simulink model "ImpMinJerkTraj"  (R2025b)
settings: Solver=FixedStepAuto  StartTime=0.0  StopTime=inf  FixedStep=Ts  RelTol=1e-3
model workspace (MAT data in the model file):
  SL_ROS_VariableLengthArrays_MaxSizes.CommonInfo.ArrayTruncateAction = 'EmitWarning'
  SL_ROS_VariableLengthArrays_MaxSizes.MsgTypeMap = containers.Map
  SL_ROS_VariableLengthArrays_MaxSizes.MsgTypeMap.serialization.keys = {'sensor_msgs/JointState'}
  SL_ROS_VariableLengthArrays_MaxSizes.MsgTypeMap.serialization.values{1}(1).PropertyName = 'effort'
  SL_ROS_VariableLengthArrays_MaxSizes.MsgTypeMap.serialization.values{1}(1).DataType = 'double'
  SL_ROS_VariableLengthArrays_MaxSizes.MsgTypeMap.serialization.values{1}(1).MaxLength = 3
  SL_ROS_VariableLengthArrays_MaxSizes.MsgTypeMap.serialization.values{1}(2).PropertyName = 'name'
  SL_ROS_VariableLengthArrays_MaxSizes.MsgTypeMap.serialization.values{1}(2).DataType = 'std_msgs/String'
  SL_ROS_VariableLengthArrays_MaxSizes.MsgTypeMap.serialization.values{1}(2).MaxLength = 16
  SL_ROS_VariableLengthArrays_MaxSizes.MsgTypeMap.serialization.values{1}(3).PropertyName = 'position'
  SL_ROS_VariableLengthArrays_MaxSizes.MsgTypeMap.serialization.values{1}(3).DataType = 'double'
  SL_ROS_VariableLengthArrays_MaxSizes.MsgTypeMap.serialization.values{1}(3).MaxLength = 3
  SL_ROS_VariableLengthArrays_MaxSizes.MsgTypeMap.serialization.values{1}(4).PropertyName = 'velocity'
  SL_ROS_VariableLengthArrays_MaxSizes.MsgTypeMap.serialization.values{1}(4).DataType = 'double'
  SL_ROS_VariableLengthArrays_MaxSizes.MsgTypeMap.serialization.values{1}(4).MaxLength = 3
  SL_ROS_VariableLengthArrays_MaxSizes.MsgTypeMap.serialization.uniformity = 0
  SL_ROS_VariableLengthArrays_MaxSizes.MsgTypeMap.serialization.keyType = 'char'
  SL_ROS_VariableLengthArrays_MaxSizes.MsgTypeMap.serialization.valueType = 'any'
values from neighbouring files (symbols this model uses):
  hiddenLayerSizeCtrl = 20    [InitMinJerkTraj.m]
  hiddenLayerSizeObsv = 5    [InitMinJerkTraj.m]
  p = 3    [InitMinJerkTraj.m]
  timePoints = [0, 12, 27, 44, 60]    [InitMinJerkTraj.m]
  torque2voltage = voltage_max ./ u_max    [InitMinJerkTraj.m]
  u_max = motor_max_torque * gear_ratio    [InitMinJerkTraj.m]
  u_min = - motor_max_torque * gear_ratio    [InitMinJerkTraj.m]
  Vctrl0 = 0.1 * randn(hiddenLayerSizeCtrl, inputLayerSizeCtrl)    [InitMinJerkTraj.m]
  Vobsv0 = 0.1 * randn(hiddenLayerSizeObsv, inputLayerSizeObsv)    [InitMinJerkTraj.m]
  wayPoints = [q1WayPoints; q2WayPoints; q3WayPoints]    [InitMinJerkTraj.m]
  Wctrl0 = 0.1 * randn(outputLayerSizeCtrl, hiddenLayerSizeCtrl)    [InitMinJerkTraj.m]
  Wobsv0 = 0.1 * randn(outputLayerSizeObsv, hiddenLayerSizeObsv)    [InitMinJerkTraj.m]
  x_hat0 = zeros(n, 1)    [InitMinJerkTraj.m]
undefined symbols (not defined in the file or in its folder): effort, effort_SL_Info, position, position_SL_Info
libraries: ros2lib x3, slpidlib x3, shareduavrstlib x1
settings Model: Creator=Asus  LastModifiedBy=Asus
settings OptimizationCC: DefaultParameterBehavior=Inlined  EnhancedBackFolding=on  PassReuseOutputArgsAs=Individual arguments  ZeroExternalMemoryAtStartup=off  ZeroInternalMemoryAtStartup=off  MaxStackSize=64  OptimizeBlockOrder=speed  DifferentSizesBufferReuse=on  OptimizationCustomize=off  EfficientTunableParamExpr=on
settings DebuggingCC: ParameterTunabilityLossMsg=error
settings SFSimCC: MATLABDynamicMemAlloc=off
settings RTWCC: SystemTargetFile=ert.tlc  HardwareBoard=Robot Operating System 2 (ROS 2)  TLCOptions="-aInlineSetEventsForThisBaseRateFcn=TLC_FALSE -aSuppressMultiTaskScheduler=TLC_FALSE  -aRateBasedStepFcn=0"  TemplateMakefile=ert_default_tmf  Toolchain=Colcon Tools  TargetLang=C++  Description=Embedded Coder
settings CodeAppCC: ForceParamTrailComments=on  IgnoreCustomStorageClasses=off  MaxIdLength=95.0  OperatorAnnotations=on  SimulinkDataObjDesc=on  SFDataObjDesc=on  InsertBlockDesc=on
settings ERTTargetCC: RootIOFormat=Structure reference  CodeInterfacePackaging=C++ class

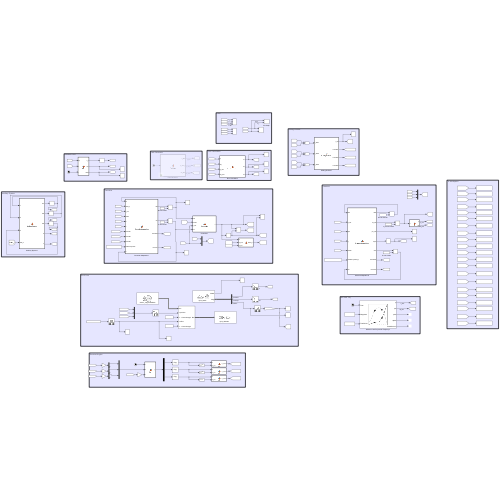
[thumbnail: Simulink's stored preview of the top-level diagram]
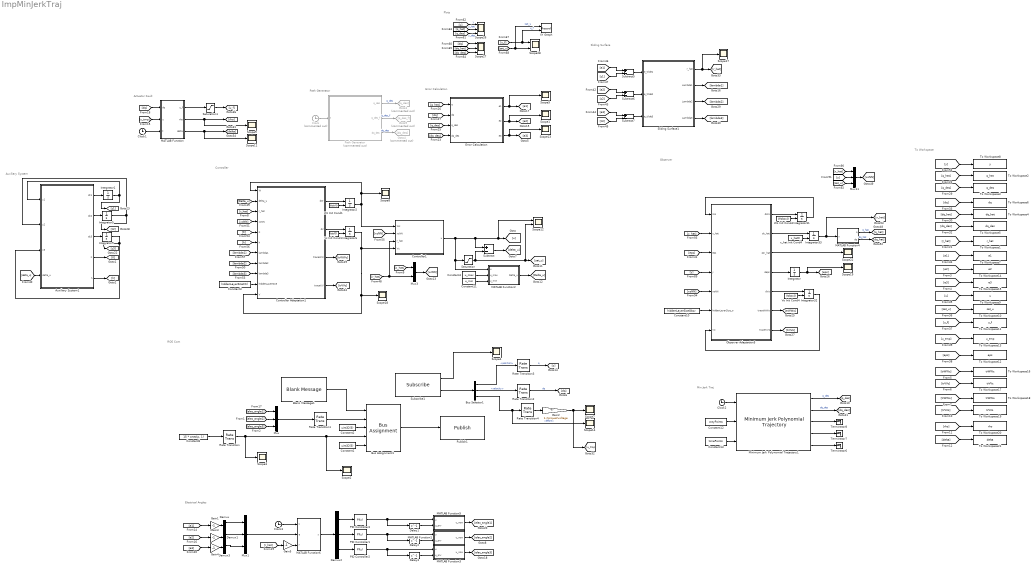
== system ImpMinJerkTraj ==
  note: To Workspace
  note: Electrical Angles
  note: Plots
  note: Path Generator
  note: Observer
  note: ROS Com
  note: Actuator Fault
  note: Min Jerk Traj
  note: Auxiliary System
  note: Error Calculation
  note: Sliding Surface
  note: Controller
  Auxiliary System1 : MATLAB Function  TreatAsAtomicUnit=on
  Blank Message1 : ros2lib/Blank Message  messageClass=Message  entityType=sensor_msgs/JointState  messageType=sensor_msgs/JointState  SampleTime=0.02
  Bus Assignment1 : BusAssignment  AssignedSignals=position,position_SL_Info.CurrentLength,effort,effort_SL_Info.CurrentLength
  Bus Selector1 : BusSelector  OutputSignals=position,velocity,effort
  Clock : Clock  Commented=on
  Clock1 : Clock
  Clock2 : Clock
  Clock3 : Clock
  Constant1 : Constant  Value=uint32(3)
  Constant10 : Constant  Value=hiddenLayerSizeObsv
  Constant11 : Constant  Value=u_min
  Constant12 : Constant  Value=wayPoints
  Constant13 : Constant  Value=timePoints
  Constant2 : Constant  Value=uint32(3)
  Constant3 : Constant  Value=hiddenLayerSizeCtrl
  Constant4 : Constant  Value=u_max
  Constant8 : Constant  Value=15 * ones(p, 1)
  Controller Adaptation1 : MATLAB Function  TreatAsAtomicUnit=on
  Controller1 : MATLAB Function  TreatAsAtomicUnit=on
  Delay1 : Delay  DelayLength=1  InitialCondition=0
  Delay2 : Delay  DelayLength=1  InitialCondition=0
  Delay3 : Delay  DelayLength=1  InitialCondition=0
  Demux : Demux  Outputs=2
  Demux1 : Demux  Outputs=2
  Demux2 : Demux  Outputs=3
  Demux3 : Demux  Outputs=2
  Error Calculation : MATLAB Function  TreatAsAtomicUnit=on
  Gain{1,3..5} (4 alike) : Gain  Gain=-1
  Gain2 : Gain  Gain=1./torque2voltage
  Goto3 : Goto  Commented=on  GotoTag=q_des
  Goto4 : Goto  Commented=on  GotoTag=dq_des
  Goto9 : Goto  Commented=on  GotoTag=q_des_f
  Integrator : Integrator  InitialCondition=5 * ones(p, 1)
  Integrator1 : Integrator  InitialCondition=zeros(2, 1)
  Integrator{2,6,31..33} (5 alike) : Integrator  InitialConditionSource=external  InitialCondition=[0.5; 0.5]
  Integrator5 : Integrator  InitialCondition=zeros(2, 1)
  Integrator9 : Integrator  InitialCondition=zeros(2, 1)
  MATLAB Function : MATLAB Function  TreatAsAtomicUnit=on
  MATLAB Function1 : MATLAB Function  TreatAsAtomicUnit=on
  MATLAB Function2 : MATLAB Function  TreatAsAtomicUnit=on
  MATLAB Function3 : MATLAB Function  TreatAsAtomicUnit=on
  MATLAB Function4 : MATLAB Function  TreatAsAtomicUnit=on
  MATLAB Function5 : MATLAB Function  TreatAsAtomicUnit=on
  MATLAB Function6 : MATLAB Function  TreatAsAtomicUnit=on
  Minimum Jerk Polynomial Trajectory1 : shareduavrstlib/Minimum Jerk Polynomial Trajectory  ShowBCInputPort=off  ShowPolynomialCoefs=off  ShowStatusOutputPort=off  TimeAllocation=off  TimeWeight=100  MinSegmentTime=0.1  MaxSegmentTime=1  MaxIteration=1500  MaxTime=10  SimulateUsing=Interpreted execution
      settings: LibrarySourceBlock=robotutilslib/Minimum Jerk Polynomial Trajectory
  Mux : Mux  Inputs=3
  Mux1 : Mux  Inputs=3
  Mux11 : Mux  Inputs=3
  Mux3 : Mux  Inputs=2
  Observer Adaptation5 : MATLAB Function  TreatAsAtomicUnit=on
  PID Controller1 : slpidlib/PID Controller  Controller=PI  Form=Parallel  TimeDomain=Discrete-time  UseExternalTs=off  SampleTime=-1  IntegratorMethod=Trapezoidal  FilterMethod=Forward Euler  ControllerParametersSource=internal  P=0.01  I=20  UseKiTs=off  D=0  UseExternalDerivativeSource=off  N=100  UseFilter=on  TunerSelectOption=Transfer Function Based (PID Tuner App)  InitialConditionSource=internal  InitialConditionForIntegrator=0  InitialConditionForFilter=0  DifferentiatorICPrevScaledInput=0  ExternalReset=none  TrackingMode=off  Kt=1  LimitOutput=off  SatLimitsSource=internal  UpperSaturationLimit=50  LowerSaturationLimit=-50  LinearizeAsGain=on  AntiWindupMode=none  Kb=1  LimitIntegrator=off  UpperIntegratorSaturationLimit=50  LowerIntegratorSaturationLimit=-50  POutMin=[]  POutMax=[]  IOutMin=[]  IOutMax=[]  DOutMin=[]  DOutMax=[]  NOutMin=[]  NOutMax=[]  SumOutMin=[]  SumOutMax=[]  SaturationOutMin=[]  SaturationOutMax=[]  PParamMin=[]  PParamMax=[]  IParamMin=[]  IParamMax=[]  DParamMin=[]  DParamMax=[]  NParamMin=[]  NParamMax=[]  KbParamMin=[]  KbParamMax=[]  KtParamMin=[]  KtParamMax=[]  KbOutMin=[]  KbOutMax=[]  KtOutMin=[]  KtOutMax=[]  IntegratorOutMin=[]  IntegratorOutMax=[]  FilterOutMin=[]  FilterOutMax=[]  SumI1OutMin=[]  SumI1OutMax=[]  SumI2OutMin=[]  SumI2OutMax=[]  SumI3OutMin=[]  SumI3OutMax=[]  SumI4OutMin=[]  SumI4OutMax=[]  SumDOutMin=[]  SumDOutMax=[]  DifferentiatorOutMin=[]  DifferentiatorOutMax=[]  FilterDiffOutCoefMin=[]  FilterDiffOutCoefMax=[]  ReciprocalOutMin=[]  ReciprocalOutMax=[]  SumDenOutMin=[]  SumDenOutMax=[]  SumNumOutMin=[]  SumNumOutMax=[]  DivideOutMin=[]  DivideOutMax=[]  UdiffTsProdOutMin=[]  UdiffTsProdOutMax=[]  NTsProdOutMin=[]  NTsProdOutMax=[]  UintegralTsProdOutMin=[]  UintegralTsProdOutMax=[]  UngainTsProdOutMin=[]  UngainTsProdOutMax=[]  ClampingZeroOutDataTypeStr=Inherit: Inherit via back propagation  ClampingZeroOutMin=[]  ClampingZeroOutMax=[]  FilterDenConstantOutDataTypeStr=Inherit: Inherit via back propagation  FilterDenConstantOutMin=[]  FilterDenConstantOutMax=[]  PCopyOutDataTypeStr=Inherit: Inherit via back propagation  PCopyOutMin=[]  PCopyOutMax=[]  NCopyOutDataTypeStr=Inherit: Inherit via back propagation  NCopyOutMin=[]  NCopyOutMax=[]  IntegratorContinuousStateAttributes=''  IntegratorStateMustResolveToSignalObject=off  IntegratorRTWStateStorageClass=Auto  FilterContinuousStateAttributes=''  FilterStateMustResolveToSignalObject=off  FilterRTWStateStorageClass=Auto  ParallelPVariant=InternalParameters  IdealPVariant=Disabled  IVariant=InternalParameters  DVariant=Disabled  IntegratorVariant=Discrete  SatVariant=Disabled  AWVariant=Passthrough  PCopyVariant=Disabled  TRVariant=Disabled  FdbkBlocksVariant=Forward  IdealPFdbkVariant=Disabled  SatFdbkVariant=Disabled  DerivativeFilterVariant=Disabled  NVariant=Disabled  NCopyVariant=Disabled_SignalSpec  FilterICVariant=Disabled  IntegratorICVariant=InternalICs  ExternalResetVariant=Disabled  TRSumVariant=Passthrough  SumFdbkVariant=Disabled  SumVariant=Sum_PI  TsampFilterVariant=InternalTs  TsampNgainVariant=Passthrough  TsampIntegralVariant=Disabled_SignalSpec  ExternalSaturationOutDataTypeStr=Inherit: Same as second input  DerivativeSourceVariant=Disabled  PreIntVariant=InternalPreInt
  PID Controller2 : slpidlib/PID Controller  Controller=PI  Form=Parallel  TimeDomain=Discrete-time  UseExternalTs=off  SampleTime=-1  IntegratorMethod=Trapezoidal  FilterMethod=Forward Euler  ControllerParametersSource=internal  P=0.01  I=20  UseKiTs=off  D=0  UseExternalDerivativeSource=off  N=100  UseFilter=on  TunerSelectOption=Transfer Function Based (PID Tuner App)  InitialConditionSource=internal  InitialConditionForIntegrator=0  InitialConditionForFilter=0  DifferentiatorICPrevScaledInput=0  ExternalReset=none  TrackingMode=off  Kt=1  LimitOutput=off  SatLimitsSource=internal  UpperSaturationLimit=50  LowerSaturationLimit=-50  LinearizeAsGain=on  AntiWindupMode=none  Kb=1  LimitIntegrator=off  UpperIntegratorSaturationLimit=50  LowerIntegratorSaturationLimit=-50  POutMin=[]  POutMax=[]  IOutMin=[]  IOutMax=[]  DOutMin=[]  DOutMax=[]  NOutMin=[]  NOutMax=[]  SumOutMin=[]  SumOutMax=[]  SaturationOutMin=[]  SaturationOutMax=[]  PParamMin=[]  PParamMax=[]  IParamMin=[]  IParamMax=[]  DParamMin=[]  DParamMax=[]  NParamMin=[]  NParamMax=[]  KbParamMin=[]  KbParamMax=[]  KtParamMin=[]  KtParamMax=[]  KbOutMin=[]  KbOutMax=[]  KtOutMin=[]  KtOutMax=[]  IntegratorOutMin=[]  IntegratorOutMax=[]  FilterOutMin=[]  FilterOutMax=[]  SumI1OutMin=[]  SumI1OutMax=[]  SumI2OutMin=[]  SumI2OutMax=[]  SumI3OutMin=[]  SumI3OutMax=[]  SumI4OutMin=[]  SumI4OutMax=[]  SumDOutMin=[]  SumDOutMax=[]  DifferentiatorOutMin=[]  DifferentiatorOutMax=[]  FilterDiffOutCoefMin=[]  FilterDiffOutCoefMax=[]  ReciprocalOutMin=[]  ReciprocalOutMax=[]  SumDenOutMin=[]  SumDenOutMax=[]  SumNumOutMin=[]  SumNumOutMax=[]  DivideOutMin=[]  DivideOutMax=[]  UdiffTsProdOutMin=[]  UdiffTsProdOutMax=[]  NTsProdOutMin=[]  NTsProdOutMax=[]  UintegralTsProdOutMin=[]  UintegralTsProdOutMax=[]  UngainTsProdOutMin=[]  UngainTsProdOutMax=[]  ClampingZeroOutDataTypeStr=Inherit: Inherit via back propagation  ClampingZeroOutMin=[]  ClampingZeroOutMax=[]  FilterDenConstantOutDataTypeStr=Inherit: Inherit via back propagation  FilterDenConstantOutMin=[]  FilterDenConstantOutMax=[]  PCopyOutDataTypeStr=Inherit: Inherit via back propagation  PCopyOutMin=[]  PCopyOutMax=[]  NCopyOutDataTypeStr=Inherit: Inherit via back propagation  NCopyOutMin=[]  NCopyOutMax=[]  IntegratorContinuousStateAttributes=''  IntegratorStateMustResolveToSignalObject=off  IntegratorRTWStateStorageClass=Auto  FilterContinuousStateAttributes=''  FilterStateMustResolveToSignalObject=off  FilterRTWStateStorageClass=Auto  ParallelPVariant=InternalParameters  IdealPVariant=Disabled  IVariant=InternalParameters  DVariant=Disabled  IntegratorVariant=Discrete  SatVariant=Disabled  AWVariant=Passthrough  PCopyVariant=Disabled  TRVariant=Disabled  FdbkBlocksVariant=Forward  IdealPFdbkVariant=Disabled  SatFdbkVariant=Disabled  DerivativeFilterVariant=Disabled  NVariant=Disabled  NCopyVariant=Disabled_SignalSpec  FilterICVariant=Disabled  IntegratorICVariant=InternalICs  ExternalResetVariant=Disabled  TRSumVariant=Passthrough  SumFdbkVariant=Disabled  SumVariant=Sum_PI  TsampFilterVariant=InternalTs  TsampNgainVariant=Passthrough  TsampIntegralVariant=Disabled_SignalSpec  ExternalSaturationOutDataTypeStr=Inherit: Same as second input  DerivativeSourceVariant=Disabled  PreIntVariant=InternalPreInt
  PID Controller4 : slpidlib/PID Controller  Controller=PI  Form=Parallel  TimeDomain=Discrete-time  UseExternalTs=off  SampleTime=-1  IntegratorMethod=Trapezoidal  FilterMethod=Forward Euler  ControllerParametersSource=internal  P=0.01  I=20  UseKiTs=off  D=0  UseExternalDerivativeSource=off  N=100  UseFilter=on  TunerSelectOption=Transfer Function Based (PID Tuner App)  InitialConditionSource=internal  InitialConditionForIntegrator=0  InitialConditionForFilter=0  DifferentiatorICPrevScaledInput=0  ExternalReset=none  TrackingMode=off  Kt=1  LimitOutput=off  SatLimitsSource=internal  UpperSaturationLimit=50  LowerSaturationLimit=-50  LinearizeAsGain=on  AntiWindupMode=none  Kb=1  LimitIntegrator=off  UpperIntegratorSaturationLimit=50  LowerIntegratorSaturationLimit=-50  POutMin=[]  POutMax=[]  IOutMin=[]  IOutMax=[]  DOutMin=[]  DOutMax=[]  NOutMin=[]  NOutMax=[]  SumOutMin=[]  SumOutMax=[]  SaturationOutMin=[]  SaturationOutMax=[]  PParamMin=[]  PParamMax=[]  IParamMin=[]  IParamMax=[]  DParamMin=[]  DParamMax=[]  NParamMin=[]  NParamMax=[]  KbParamMin=[]  KbParamMax=[]  KtParamMin=[]  KtParamMax=[]  KbOutMin=[]  KbOutMax=[]  KtOutMin=[]  KtOutMax=[]  IntegratorOutMin=[]  IntegratorOutMax=[]  FilterOutMin=[]  FilterOutMax=[]  SumI1OutMin=[]  SumI1OutMax=[]  SumI2OutMin=[]  SumI2OutMax=[]  SumI3OutMin=[]  SumI3OutMax=[]  SumI4OutMin=[]  SumI4OutMax=[]  SumDOutMin=[]  SumDOutMax=[]  DifferentiatorOutMin=[]  DifferentiatorOutMax=[]  FilterDiffOutCoefMin=[]  FilterDiffOutCoefMax=[]  ReciprocalOutMin=[]  ReciprocalOutMax=[]  SumDenOutMin=[]  SumDenOutMax=[]  SumNumOutMin=[]  SumNumOutMax=[]  DivideOutMin=[]  DivideOutMax=[]  UdiffTsProdOutMin=[]  UdiffTsProdOutMax=[]  NTsProdOutMin=[]  NTsProdOutMax=[]  UintegralTsProdOutMin=[]  UintegralTsProdOutMax=[]  UngainTsProdOutMin=[]  UngainTsProdOutMax=[]  ClampingZeroOutDataTypeStr=Inherit: Inherit via back propagation  ClampingZeroOutMin=[]  ClampingZeroOutMax=[]  FilterDenConstantOutDataTypeStr=Inherit: Inherit via back propagation  FilterDenConstantOutMin=[]  FilterDenConstantOutMax=[]  PCopyOutDataTypeStr=Inherit: Inherit via back propagation  PCopyOutMin=[]  PCopyOutMax=[]  NCopyOutDataTypeStr=Inherit: Inherit via back propagation  NCopyOutMin=[]  NCopyOutMax=[]  IntegratorContinuousStateAttributes=''  IntegratorStateMustResolveToSignalObject=off  IntegratorRTWStateStorageClass=Auto  FilterContinuousStateAttributes=''  FilterStateMustResolveToSignalObject=off  FilterRTWStateStorageClass=Auto  ParallelPVariant=InternalParameters  IdealPVariant=Disabled  IVariant=InternalParameters  DVariant=Disabled  IntegratorVariant=Discrete  SatVariant=Disabled  AWVariant=Passthrough  PCopyVariant=Disabled  TRVariant=Disabled  FdbkBlocksVariant=Forward  IdealPFdbkVariant=Disabled  SatFdbkVariant=Disabled  DerivativeFilterVariant=Disabled  NVariant=Disabled  NCopyVariant=Disabled_SignalSpec  FilterICVariant=Disabled  IntegratorICVariant=InternalICs  ExternalResetVariant=Disabled  TRSumVariant=Passthrough  SumFdbkVariant=Disabled  SumVariant=Sum_PI  TsampFilterVariant=InternalTs  TsampNgainVariant=Passthrough  TsampIntegralVariant=Disabled_SignalSpec  ExternalSaturationOutDataTypeStr=Inherit: Same as second input  DerivativeSourceVariant=Disabled  PreIntVariant=InternalPreInt
  Path Generator : MATLAB Function  Commented=on  TreatAsAtomicUnit=on
  Publish1 : ros2lib/Publish  topicSource=Specify your own  topic=/joint_desireds  messageType=sensor_msgs/JointState  QOSHistory=Keep last  QOSDepth=10  QOSReliability=Reliable  QOSDurability=Volatile  QOSDeadline=Inf  QOSLifespan=Inf  QOSLiveliness=Automatic  QOSLeaseDuration=Inf  QOSAvoidROSNamespaceConventions=off
  Rate Transition : RateTransition  OutPortSampleTime=0.02
  Rate Transition1 : RateTransition  OutPortSampleTime=0.02
  Rate Transition2 : RateTransition  OutPortSampleTime=Ts
  Rate Transition3 : RateTransition  OutPortSampleTime=Ts
  Rate Transition4 : RateTransition  OutPortSampleTime=Ts
  Saturation : Saturate  UpperLimit=u_max  LowerLimit=u_min
  Saturation1 : Saturate  UpperLimit=u_max  LowerLimit=u_min
  Scope{1..5,7..9,11,13..14,17..19,22} (15 alike) : Scope
      Scope1 settings: ActiveDisplayYMinimum=-0.24287807344006263  ActiveDisplayYMaximum=0.25287974310957717  DataLoggingVariableName=ScopeData3
      Scope11 settings: ActiveDisplayYMinimum=-1  ActiveDisplayYMaximum=1  DataLoggingVariableName=ScopeData6
      Scope13 settings: ActiveDisplayYMinimum=-0.29897924911149121  ActiveDisplayYMaximum=0.2090765790905024  DataLoggingVariableName=ScopeData13
      Scope14 settings: ActiveDisplayYMinimum=-12.649985074996948  ActiveDisplayYMaximum=12.652279615402222  DataLoggingVariableName=ScopeData14
      Scope17 settings: ActiveDisplayYMinimum=-9.1334368109122082  ActiveDisplayYMaximum=5.1770184739117182  DataLoggingVariableName=ScopeData19
      Scope18 settings: ActiveDisplayYMinimum=-1  ActiveDisplayYMaximum=1  DataLoggingVariableName=ScopeData10
      Scope19 settings: ActiveDisplayYMinimum=-0.056716812017258533  ActiveDisplayYMaximum=20.510451308155332  DataLoggingVariableName=ScopeData15
      Scope2 settings: ActiveDisplayYMinimum=-1.8749999999999996  ActiveDisplayYMaximum=16.875
      Scope22 settings: ActiveDisplayYMinimum=-0.42606678523590263  ActiveDisplayYMaximum=0.48150686097965856  DataLoggingVariableName=ScopeData18
      Scope3 settings: ActiveDisplayYMinimum=5  ActiveDisplayYMaximum=25  DataLoggingVariableName=ScopeData4
      Scope4 settings: ActiveDisplayYMinimum=-0.12499999999999997  ActiveDisplayYMaximum=1.125  DataLoggingVariableName=ScopeData11
      Scope5 settings: ActiveDisplayYMinimum=-0.20021441252280484  ActiveDisplayYMaximum=0.22401805193004884
      Scope7 settings: ActiveDisplayYMinimum=-9.2534578715761491  ActiveDisplayYMaximum=9.2113278185327836  DataLoggingVariableName=ScopeData8
      Scope8 settings: ActiveDisplayYMinimum=-68.998192796896234  ActiveDisplayYMaximum=67.9276309158068  DataLoggingVariableName=ScopeData20
      Scope9 settings: ActiveDisplayYMinimum=0.62111967257868006  ActiveDisplayYMaximum=1.4258213646991535  DataLoggingVariableName=ScopeData5
  Scope12 : Scope  NumInputPorts=2
      settings: ActiveDisplayYMinimum=-7.8125  ActiveDisplayYMaximum=7.8125  DataLoggingVariableName=ScopeData7
  Scope26 : Scope  NumInputPorts=3
      settings: ActiveDisplayYMinimum=-0.93551342302711427  ActiveDisplayYMaximum=1.30254068575359  DataLoggingVariableName=ScopeData22
  Scope27 : Scope  NumInputPorts=3
      settings: ActiveDisplayYMinimum=-14.15664383431546  ActiveDisplayYMaximum=27.525156502809544  DataLoggingVariableName=ScopeData23
  Scope28 : Scope  NumInputPorts=2
      settings: ActiveDisplayYMinimum=-9.023426901335915  ActiveDisplayYMaximum=9.2220209186866775  DataLoggingVariableName=ScopeData24
  Sliding Surface1 : MATLAB Function  TreatAsAtomicUnit=on
  Subscribe1 : ros2lib/Subscribe  topicSource=Select from ROS network  topic=/joint_states  messageType=sensor_msgs/JointState  sampleTime=0.02  QOSHistory=Keep all  QOSDepth=3  QOSReliability=Best effort  QOSDurability=Volatile  QOSDeadline=Inf  QOSLifespan=Inf  QOSLiveliness=Automatic  QOSLeaseDuration=Inf  QOSAvoidROSNamespaceConventions=off
  Subtract{,5..7} (4 alike) : Sum  Inputs=+-
  Terminator6 : Terminator
  Terminator7 : Terminator
  Terminator8 : Terminator
  To Workspace1 : ToWorkspace  VariableName=r_hat  SaveFormat=Structure  SampleTime=-1
      settings: Save2DSignal=2-D array (concatenate along first dimension)
  To Workspace10 : ToWorkspace  VariableName=sat_u  SaveFormat=Structure  SampleTime=-1
      settings: Save2DSignal=2-D array (concatenate along first dimension)
  To Workspace11 : ToWorkspace  VariableName=u_f  SaveFormat=Structure  SampleTime=-1
      settings: Save2DSignal=2-D array (concatenate along first dimension)
  To Workspace12 : ToWorkspace  VariableName=eps  SaveFormat=Structure  SampleTime=-1
      settings: Save2DSignal=2-D array (concatenate along first dimension)
  To Workspace13 : ToWorkspace  VariableName=u_tmp  SaveFormat=Structure  SampleTime=-1
      settings: Save2DSignal=2-D array (concatenate along first dimension)
  To Workspace14 : ToWorkspace  VariableName=e2  SaveFormat=Structure  SampleTime=-1
      settings: Save2DSignal=2-D array (concatenate along first dimension)
  To Workspace15 : ToWorkspace  VariableName=e3  SaveFormat=Structure  SampleTime=-1
      settings: Save2DSignal=2-D array (concatenate along first dimension)
  To Workspace16 : ToWorkspace  VariableName=trWWc  SaveFormat=Structure  SampleTime=-1
      settings: Save2DSignal=2-D array (concatenate along first dimension)
  To Workspace17 : ToWorkspace  VariableName=trVVc  SaveFormat=Structure  SampleTime=-1
      settings: Save2DSignal=2-D array (concatenate along first dimension)
  To Workspace18 : ToWorkspace  VariableName=trWWo  SaveFormat=Structure  SampleTime=-1
      settings: Save2DSignal=2-D array (concatenate along first dimension)
  To Workspace19 : ToWorkspace  VariableName=trVVo  SaveFormat=Structure  SampleTime=-1
      settings: Save2DSignal=2-D array (concatenate along first dimension)
  To Workspace2 : ToWorkspace  VariableName=q_hat  SaveFormat=Structure  SampleTime=-1
      settings: Save2DSignal=2-D array (concatenate along first dimension)
  To Workspace20 : ToWorkspace  VariableName=rho  SaveFormat=Structure  SampleTime=-1
      settings: Save2DSignal=2-D array (concatenate along first dimension)
  To Workspace21 : ToWorkspace  VariableName=delta  SaveFormat=Structure  SampleTime=-1
      settings: Save2DSignal=2-D array (concatenate along first dimension)
  To Workspace3 : ToWorkspace  VariableName=q_des  SaveFormat=Structure  SampleTime=-1
      settings: Save2DSignal=2-D array (concatenate along first dimension)
  To Workspace4 : ToWorkspace  VariableName=dq_hat  SaveFormat=Structure  SampleTime=-1
      settings: Save2DSignal=2-D array (concatenate along first dimension)
  To Workspace5 : ToWorkspace  VariableName=dq_des  SaveFormat=Structure  SampleTime=-1
      settings: Save2DSignal=2-D array (concatenate along first dimension)
  To Workspace6 : ToWorkspace  VariableName=dq  SaveFormat=Structure  SampleTime=-1
      settings: Save2DSignal=2-D array (concatenate along first dimension)
  To Workspace7 : ToWorkspace  VariableName=e1  SaveFormat=Structure  SampleTime=-1
      settings: Save2DSignal=2-D array (concatenate along first dimension)
  To Workspace8 : ToWorkspace  VariableName=y  SaveFormat=Structure  SampleTime=-1
      settings: Save2DSignal=2-D array (concatenate along first dimension)
  To Workspace9 : ToWorkspace  VariableName=u  SaveFormat=Structure  SampleTime=-1
      settings: Save2DSignal=2-D array (concatenate along first dimension)
  Vc Init Cond1 : Constant  Value=Vctrl0
  Vo Init Cond4 : Constant  Value=Vobsv0
  Wc Init Cond1 : Constant  Value=Wctrl0
  Wo Init Cond4 : Constant  Value=Wobsv0
  XY Graph : Record  NumPorts=2.0  FileSettingsInternal="{\"entries\":[{\"content\":{\"excelSettings\":{\"content\":{},\"type\":\"Streamout.ExcelSettings\"},\"parquetSettings\":{\"content\":{},\"type\":\"Streamout.ParquetSettings\"}},\"type\":\"Streamout.FileSettingStorage\",\"uuid\":\"\"}],\"packageUris\":[\"http:\\/\\/schema.mathworks.com\\/mf0\\/streamout_blocks\\/R2020a\"],\"version\":\"1.0\"}"  FrameSettings=[0, 0]  Layout=[1 1]  SignalsInternal="{\"entries\":[{\"content\":{\"signals\":[{\"content\":{\"blockPath\":[],\"dimensions\":[3,1],\"domain\":\"\",\"hasChildren\":true,\"lineColor\":\"#77ac30\",\"lineWidth\":2,\"port\":1,\"sid\":[\"\"],\"signalID\":1,\"signalName\":\"sat_u\"},\"type\":\"RecordBlkView.Signal\",\"uuid\":\"\"},{\"content\":{\"blockPath\":[],\"channel\":[1,1],\"dimensions\":[3,1],\"domain\":\"\",\"lineColor\":\"#64d413\",\"lineWidth\":2,\"parentID\":1,\"port\":1,\"sid\":[\"\"],\"signalID\":2,\"signalName\":\"sat_u\"},\"type\":\"RecordBlkView.Signal\",\"uuid\":\"\"},{\"content\":{\"blockPath\":[],\"dimensions\":[3,1],\"domain\":\"\",\"hasChildren\":true,\"lineColor\":\"#a2142f\",\"lineWidth\":2,\"port\":2,\"sid\":[\"\"],\"signalID\":3,\"signalName\":\"u_f\"},\"type\":\"RecordBlkView.Signal\",\"uuid\":\"\"},{\"content\":{\"blockPath\":[],\"channel\":[1,1],\"dimensions\":[3,1],\"domain\":\"\",\"lineColor\":\"#fe330a\",\"lineWidth\":2,\"parentID\":3,\"port\":2,\"sid\":[\"\"],\"signalID\":4,\"signalName\":\"u_f\"},\"type\":\"RecordBlkView.Signal\",\"uuid\":\"\"},{\"content\":{\"blockPath\":[],\"channel\":[2,1],\"dimensions\":[3,1],\"domain\":\"\",\"lineColor\":\"#d95319\",\"lineWidth\":2,\"parentID\":1,\"plots\":[ 1 ],\"port\":1,\"sid\":[\"\"],\"signalID\":5,\"signalName\":\"sat_u\"},\"type\":\"RecordBlkView.Signal\",\"uuid\":\"\"},{\"content\":{\"blockPath\":[],\"channel\":[3,1],\"dimensions\":[3,1],\"domain\":\"\",\"lineColor\":\"#edb120\",\"lineWidth\":2,\"parentID\":1,\"port\":1,\"sid\":[\"\"],\"signalID\":6,\"signalName\":\"sat_u\"},\"type\":\"RecordBlkView.Signal\",\"uuid\":\"\"},{\"content\":{\"blockPath\":[],\"channel\":[2,1],\"dimensions\":[3,1],\"domain\":\"\",\"lineColor\":\"#7e2f8e\",\"lineWidth\":2,\"parentID\":3,\"plots\":[ 1 ],\"port\":2,\"sid\":[\"\"],\"signalID\":7,\"signalName\":\"u_f\"},\"type\":\"RecordBlkView.Signal\",\"uuid\":\"\"},{\"content\":{\"blockPath\":[],\"channel\":[3,1],\"dimensions\":[3,1],\"domain\":\"\",\"lineColor\":\"#77ac30\",\"lineWidth\":2,\"parentID\":3,\"port\":2,\"sid\":[\"\"],\"signalID\":8,\"signalName\":\"u_f\"},\"type\":\"RecordBlkView.Signal\",\"uuid\":\"\"}]},\"type\":\"RecordBlkView.InputSignals\",\"uuid\":\"\"}],\"packageUris\":[\"http:\\/\\/schema.mathworks.com\\/mf0\\/streamout_blocks\\/R2020a\"],\"version\":\"1.0\"}"  VisualizationBindings="{\"xyplotplugin\":{\"info\":[{\"series\":[{\"bindingParametersList\":[{\"parameter\":\"X-Axis\",\"signalID\":5,\"signalName\":\"sat_u(2,1)\"},{\"parameter\":\"Y-Axis\",\"signalID\":7,\"signalName\":\"u_f(2,1)\"}],\"seriesID\":0}],\"subplotID\":1}]}}"  CompatibilityTag=XY
  x_hat Init Cond4 : Constant  Value=x_hat0
  wires:
  Mux/1 -> Rate Transition1/1
  Blank Message1/1 -> Bus Assignment1/1
  Integrator31/1 -> Observer Adaptation5/1(Wo)
  Wo Init Cond4/1 -> Integrator31/2
  Bus Selector1/2 -> Rate Transition2/1  "<velocity>"
  Observer Adaptation5/4(deps) -> Integrator/1
  Vo Init Cond4/1 -> Integrator32/2
  [x_hat] -> Observer Adaptation5/2(x_hat)
  [dq] -> MATLAB Function/1(dq)
  Bus Assignment1/1 -> Publish1/1
  MATLAB Function/2(rho) -> [rho], Scope9/1
  Path Generator/1(q_des) -> Goto3/1  "q_des"
  [y] -> Observer Adaptation5/4(y)
  MATLAB Function/3(delta) -> [delta], Scope11/1
  [eps] -> Observer Adaptation5/3(eps)
  [sat_u] -> Mux11/3
  Clock1/1 -> MATLAB Function/3(t)
  [dq_des] -> Scope27/3
  MATLAB Function4/1(q) -> [q_hat]  "q_hat"
  [u_tmp] -> MATLAB Function/2(u)
  Bus Selector1/1 -> Rate Transition3/1  "<position>"
  [q_des] -> Scope26/3  "y_des"
  Rate Transition1/1 -> Bus Assignment1/2
  Observer Adaptation5/1(dWo) -> Integrator31/1
  Constant1/1 -> Bus Assignment1/5
  MATLAB Function/1(u_f) -> Saturation1/1
  Constant10/1 -> Observer Adaptation5/6(hiddenLayerSize_o)
  [x_hat] -> Mux11/1
  [y] -> Mux11/2
  Integrator/1 -> Scope19/1, [eps]
  Observer Adaptation5/2(dx_hat) -> Integrator33/1
  Integrator32/1 -> Observer Adaptation5/7(Vo)
  MATLAB Function4/2(dq) -> [dq_hat]  "dq_hat"
  Subscribe1/1 -> Scope4/1
  [dq] -> Scope27/1
  [q_hat] -> Scope26/2  "y_hat"
  [u_f] -> XY Graph/2, Scope28/1  "u_f"
  [dq_hat] -> Scope27/2
  Clock/1 -> Path Generator/1(t)
  Subscribe1/2 -> Bus Selector1/1
  [xoNN] -> Observer Adaptation5/5(xoNN)
  x_hat Init Cond4/1 -> Integrator33/2
  [y] -> Scope26/1  "y"
  Observer Adaptation5/3(psi_hat) -> Scope22/1
  Saturation1/1 -> [u_f]
  [sat_u] -> XY Graph/1, Scope28/2  "sat_u"
  Mux11/1 -> [xoNN]
  Rate Transition4/1 -> Gain2/1
  Observer Adaptation5/5(dVo) -> Integrator32/1
  Path Generator/3(dq_des) -> Goto4/1  "dq_des"
  Bus Selector1/3 -> Scope14/1, Rate Transition4/1  "<effort>"
  Constant2/1 -> Bus Assignment1/3
  Path Generator/2(q_des_f) -> Goto9/1  "q_des_f"
  Integrator33/1 -> MATLAB Function4/1(x), [x_hat]
  Gain2/1 -> [u_tmp], Scope7/1
  Rate Transition/1 -> Scope2/1, Bus Assignment1/4, Scope3/1
  Delay1/1 -> MATLAB Function5/2(u_prv)
  MATLAB Function5/1(u_now) -> [elec_angle1]
  PID Controller4/1 -> Delay1/1, MATLAB Function5/1(u)
  [y] -> To Workspace8/1
  [r_hat] -> To Workspace1/1
  [q_hat] -> To Workspace2/1
  [q_des] -> To Workspace3/1
  [dq_hat] -> To Workspace4/1
  [dq] -> To Workspace6/1
  [dq_des] -> To Workspace5/1
  [e1] -> To Workspace7/1
  [u] -> To Workspace9/1
  [sat_u] -> To Workspace10/1
  [u_f] -> To Workspace11/1
  [eps] -> To Workspace12/1
  [u_tmp] -> To Workspace13/1
  Minimum Jerk Polynomial Trajectory1/4 -> Terminator7/1
  Constant13/1 -> Minimum Jerk Polynomial Trajectory1/3
  Constant12/1 -> Minimum Jerk Polynomial Trajectory1/2
  Minimum Jerk Polynomial Trajectory1/5 -> Terminator6/1
  Clock2/1 -> Minimum Jerk Polynomial Trajectory1/1
  Minimum Jerk Polynomial Trajectory1/2 -> [dq_des]  "dq_des"
  Minimum Jerk Polynomial Trajectory1/1 -> [q_des]  "q_des"
  Minimum Jerk Polynomial Trajectory1/3 -> Terminator8/1
  Auxiliary System1/1(dz1) -> Integrator1/1
  Auxiliary System1/3(dz3) -> Integrator9/1
  Auxiliary System1/2(dz2) -> Integrator5/1
  Integrator5/1 -> [z2], Auxiliary System1/2(z2)
  Auxiliary System1/5(h) -> [h]
  Integrator9/1 -> Auxiliary System1/3(z3), [z3]
  [delta_u] -> Auxiliary System1/4(delta_u)
  Integrator1/1 -> [z1], Auxiliary System1/1(z1)
  Auxiliary System1/4(K) -> [K]
  Error Calculation/2(e2) -> [e2], Scope1/1
  Error Calculation/1(e1) -> [e1], Scope5/1
  Error Calculation/3(e3) -> Scope13/1, [e3]
  [dq] -> Error Calculation/2(dq)
  [dq_des] -> Error Calculation/4(dq_des)
  [q_hat] -> Error Calculation/1(q)
  [q_des] -> Error Calculation/3(q_des)
  [z1] -> Subtract5/2
  Subtract6/1 -> Sliding Surface1/2(e_tilde2)
  [z3] -> Subtract7/2
  Sliding Surface1/3(Lambda2) -> [lambda2]
  Sliding Surface1/4(Lambda3) -> [lambda3]
  Sliding Surface1/2(Lambda1) -> [lambda1]
  Subtract7/1 -> Sliding Surface1/3(e_tilde3)
  Subtract5/1 -> Sliding Surface1/1(e_tilde1)
  Sliding Surface1/1(r_hat) -> Scope17/1, [r_hat]
  [e3] -> Subtract7/1
  [e1] -> Subtract5/1
  [e2] -> Subtract6/1
  [z2] -> Subtract6/2
  [r_hat] -> Controller Adaptation1/3(r_hat)
  Controller Adaptation1/2(dV) -> Integrator6/1
  MATLAB Function2/1(Delta_u) -> [Delta_u]
  Integrator2/1 -> Controller1/1(Wc), Scope8/1, Controller Adaptation1/1(W)
  [lambda3] -> Controller Adaptation1/9(lambda3)
  [xcNN] -> Controller Adaptation1/4(xcNN)
  Controller Adaptation1/1(dW) -> Integrator2/1
  Constant4/1 -> MATLAB Function2/2(u_max)
  [lambda2] -> Controller Adaptation1/8(lambda2)
  [r_hat] -> Controller1/3(r_hat), Mux3/2
  [Delta_u] -> Controller Adaptation1/2(delta_u)
  Constant11/1 -> MATLAB Function2/3(u_min)
  [lambda1] -> Controller Adaptation1/7(lambda1)
  Wc Init Cond1/1 -> Integrator2/2
  Subtract/1 -> [delta_u]
  [h] -> Controller Adaptation1/6(h)
  Vc Init Cond1/1 -> Integrator6/2
  Mux3/1 -> [xcNN]
  [xcNN] -> Controller1/2(xcNN)
  Controller1/1(u) -> Scope12/1, [u], Subtract/1, MATLAB Function2/1(u), Saturation/1
  [x_hat] -> Mux3/1
  [K] -> Controller Adaptation1/5(K)
  Constant3/1 -> Controller Adaptation1/10(hiddenLayerSize)
  Integrator6/1 -> Scope18/1, Controller Adaptation1/11(V), Controller1/4(Vc)
  Saturation/1 -> Scope12/2, [sat_u], Subtract/2
  PID Controller1/1 -> Delay2/1, MATLAB Function1/1(u)
  MATLAB Function1/1(u_now) -> [elec_angle2]
  Delay2/1 -> MATLAB Function1/2(u_prv)
  PID Controller2/1 -> Delay3/1, MATLAB Function3/1(u)
  MATLAB Function3/1(u_now) -> [elec_angle3]
  Delay3/1 -> MATLAB Function3/2(u_prv)
  [elec_angle3] -> Mux/3
  [elec_angle2] -> Mux/2
  [e2] -> To Workspace14/1
  [e3] -> To Workspace15/1
  Rate Transition3/1 -> [y]  "q"
  Rate Transition2/1 -> [dq]  "dq"
  Controller Adaptation1/3(traceWW) -> [trWWc]
  Controller Adaptation1/4(traceVV) -> [trVVc]
  Observer Adaptation5/6(traceWWo) -> [trWWo]
  Observer Adaptation5/7(traceVVo) -> [trVVo]
  [trWWc] -> To Workspace16/1
  [trVVc] -> To Workspace17/1
  [trVVo] -> To Workspace19/1
  [trWWo] -> To Workspace18/1
  [rho] -> To Workspace20/1
  [delta] -> To Workspace21/1
  [elec_angle1] -> Mux/1
  Constant8/1 -> Rate Transition/1
  Demux2/1 -> PID Controller4/1
  Demux2/2 -> PID Controller1/1
  Demux2/3 -> PID Controller2/1
  Clock3/1 -> MATLAB Function6/1(t)
  [r_hat] -> Gain5/1
  Gain5/1 -> MATLAB Function6/3(r)
  [e1] -> Gain1/1
  Gain4/1 -> Demux3/1
  Gain1/1 -> Demux/1
  [e2] -> Gain3/1
  [e3] -> Gain4/1
  Demux/1 -> Mux1/1
  Demux3/1 -> Mux1/3
  Gain3/1 -> Demux1/1
  Demux1/1 -> Mux1/2
  Mux1/1 -> MATLAB Function6/2(e)
  MATLAB Function6/1(y) -> Demux2/1

== matlab function ImpMinJerkTraj/MATLAB Function1 ==
  data: u input; u_now output; u_prv input
function u_now = fcn(u, u_prv)
    
    Ts = 1e-3;
    ramp = 50;
    output_rate = (u - u_prv) / Ts;
    u_now = u;
    
    if output_rate > ramp
		u_now = u_prv + ramp * Ts;
    end
	
    if output_rate < - ramp
		u_now = u_prv - ramp * Ts;
    end

end

== matlab function ImpMinJerkTraj/MATLAB Function3 ==
  data: u input; u_now output; u_prv input
function u_now = fcn(u, u_prv)
    
    Ts = 1e-3;
    ramp = 50;
    output_rate = (u - u_prv) / Ts;
    u_now = u;
    
    if output_rate > ramp
		u_now = u_prv + ramp * Ts;
    end
	
    if output_rate < - ramp
		u_now = u_prv - ramp * Ts;
    end

end

== matlab function ImpMinJerkTraj/Controller Adaptation1 ==
  data: dW output; dV output; W input; delta_u input; r_hat input; xcNN input; K input; h input; lambda1 input; lambda2 input; lambda3 input; hiddenLayerSize input; V input; traceWW output; traceVV output
function [dW, dV, traceWW, traceVV] = ControllerAdaptation(W, delta_u, r_hat, xcNN, K, h, lambda1, lambda2, lambda3, hiddenLayerSize, V)
    
    Sigma = @(z) (-1 + 2 ./ (1 + exp(-2 * z)));


    l = [2; 2; 2];

    A1 = [0, 1; 0, 0];
    A2 = [0, 1; 0, 0];
    A3 = [0, 1; 0, 0];

    B1 = [0; 1];
    B2 = [0; 1];
    B3 = [0; 1];

    Ac1 = A1 - B1 * ([lambda1', 1] * l(1) + [0, lambda1']);
    Ac2 = A2 - B2 * ([lambda2', 1] * l(2) + [0, lambda2']);
    Ac3 = A3 - B3 * ([lambda3', 1] * l(3) + [0, lambda3']);

    Ac = blkdiag(Ac1, Ac2, Ac3);
    B  = blkdiag(B1, B2, B3);

    eta   = 10 * [0.1, 0.1];
    gamma = [0.0001, 0.0001];

    PI_c      = diag(Sigma(V * xcNN).^2);
    PI_lambda = blkdiag([lambda1', 1], [lambda2', 1], [lambda3', 1]);
    
    dW = eta(1) * (r_hat' * PI_lambda * (-Ac^(-1) * B + K^(-1) * h * diag(delta_u)))' * Sigma(V * xcNN)' - gamma(1) * norm(r_hat) * W;
    dV = eta(2) * (r_hat' * PI_lambda * (-Ac^(-1) * B + K^(-1) * h * diag(delta_u)) * W * (eye(20) - PI_c))' * xcNN' - gamma(2) * norm(r_hat) * V;

    traceWW = trace(W' * W);
    traceVV = trace(V' * V);

end

== matlab function ImpMinJerkTraj/MATLAB Function6 ==
  data: t input; y output; e input; r input
function y = fcn(t, e, r)

    t0 = 0;

    if t < t0
        y = r;
    else
        y = e;
    end

end

== matlab function ImpMinJerkTraj/Error Calculation ==
  data: e1 output; e2 output; q input; dq input; q_des input; dq_des input; e3 output
function [e1, e2, e3] = ErrorCalculation(q, dq, q_des, dq_des)

    % e1 = zeros(2, 1);
    % e2 = zeros(2, 1);
    % e3 = zeros(2, 1);

    y_bar1 = [q(1); dq(1)];
    y_bar2 = [q(2); dq(2)];
    y_bar3 = [q(3); dq(3)];

    y_bar_des1 = [q_des(1); dq_des(1)];
    y_bar_des2 = [q_des(2); dq_des(2)];
    y_bar_des3 = [q_des(3); dq_des(3)];

    e1 = y_bar1 - y_bar_des1;
    e2 = y_bar2 - y_bar_des2;
    e3 = y_bar3 - y_bar_des3;
    
end

== matlab function ImpMinJerkTraj/Auxiliary System1 ==
  data: z1 input; z2 input; z3 input; dz1 output; delta_u input; dz2 output; dz3 output; K output; h output
function [dz1, dz2, dz3, K, h] = AuxiliarySystem(z1, z2, z3, delta_u)
    
    K1  = 1000 * diag([-1, -2]); K2  = 1000 * diag([-1, -2]); K3  = 1000 * diag([-1, -2]);
    h1  = - 5 * [-1; -1]; h2  = - 5 * [-1; -1]; h3  = - 5 * [-1; -1];
    
    K = blkdiag(K1, K2, K3);
    h = blkdiag(h1, h2, h3);

    dz1 = K1 * z1 + h1 * delta_u(1);
    dz2 = K2 * z2 + h2 * delta_u(2);
    dz3 = K3 * z3 + h3 * delta_u(3);
    
end

== matlab function ImpMinJerkTraj/MATLAB Function5 ==
  data: u input; u_now output; u_prv input
function u_now = fcn(u, u_prv)
    
    Ts = 1e-3;
    ramp = 50;
    output_rate = (u - u_prv) / Ts;
    u_now = u;
    
    if output_rate > ramp
		u_now = u_prv + ramp * Ts;
    end
	
    if output_rate < - ramp
		u_now = u_prv - ramp * Ts;
    end

end

== matlab function ImpMinJerkTraj/Controller1 ==
  data: u output; Wc input; xcNN input; r_hat input; Vc input
function u = Controller(Wc, xcNN, r_hat, Vc)

    Sigma = @(z) (-1 + 2 ./ (1 + exp(-2 * z)));

    K   = 0 * diag([1, 1, 1]);

    u = - Wc * Sigma(Vc * xcNN) - K * r_hat;
    
end

== matlab function ImpMinJerkTraj/MATLAB Function2 ==
  data: u input; Delta_u output; u_max input; u_min input
function Delta_u = fcn(u, u_max, u_min)

    Delta_u = zeros(3, 1);
    for i = 1:3
        if u(i) > u_max(i)
            Delta_u(i)   = 1;
        elseif u(i) < u_min(i)
            Delta_u(i)   = 1;
        else
            Delta_u(i)   = 0;
        end
    end

end

== matlab function ImpMinJerkTraj/MATLAB Function4 ==
  data: x input; q output; dq output
function [q, dq] = fcn(x)

    q  = x([1, 3, 5]);
    dq = x([2, 4, 6]);

end

== matlab function ImpMinJerkTraj/Observer Adaptation5 ==
  data: dWo output; dx_hat output; psi_hat output; deps output; dVo output; Wo input; x_hat input; eps input; y input; xoNN input; hiddenLayerSize_o input; Vo input; traceWWo output; traceVVo output
function [dWo, dx_hat, psi_hat, deps, dVo, traceWWo, traceVVo] = ObserverAdaptation(Wo, x_hat, eps, y, xoNN, hiddenLayerSize_o, Vo)

    Sigma = @(z) (-1 + 2 ./ (1 + exp(-2 * z)));
    Sigma_o = Sigma(Vo * xoNN);


    B1    = [0; 1]; B2 = [0; 1]; B3 = [0; 1];
    C1    = [1; 0]; C2 = [1; 0]; C3 = [1; 0];

    B     = blkdiag(B1, B2, B3);
    C     = blkdiag(C1, C2, C3);
    
    A1 = [0, 1; 0, 0];
    A2 = [0, 1; 0, 0];
    A3 = [0, 1; 0, 0];
    A  = blkdiag(A1, A2, A3);

    y_hat   = C' * x_hat;
    y_tilde = y - y_hat;

    alpha  = [2, 10; 2, 10; 2, 10];
    lambda = [0.01; 0.01; 0.01];
    kappa  = 100 ./ lambda;
    deps   = zeros(3, 1);
    for i  = 1:3
        if abs(y_tilde(i)) > lambda(i)
            deps(i) = kappa(i) * y_tilde(i)^2;
        end
    end
    
    rho1 = 2; rho2 = 2; rho3 = 2;
    Ho = diag([alpha(1, 2)*eps(1)^rho1; alpha(2, 2)*eps(2)^rho2; alpha(3, 2)*eps(3)^rho3]);
    
    D1 = [alpha(1, 1)*eps(1); 0]; D2 = [alpha(2, 1)*eps(2); 0]; D3 = [alpha(3, 1)*eps(3); 0];
    D  = blkdiag(D1, D2, D3);

    Ao   = A  - D*C';
    Aocl = Ao - B*Ho*C';

    psi_hat = Wo * Sigma_o;
    dx_hat  = Ao * x_hat + B * (psi_hat + Ho * y_tilde) + D * y;

    eta_o   = 5 * [10, 10];
    gamma_o = 1 * [0.01, 0.01];

    PI_o = diag(Sigma_o.^2);

    dWo = - eta_o(1) * (y_tilde' * C' * Aocl^(-1) * B)' * Sigma_o' - gamma_o(1) * norm(y_tilde) * Wo;
    dVo = - eta_o(2) * (y_tilde' * C' * Aocl^(-1) * B * Wo * (eye(5) - PI_o))' * xoNN' - gamma_o(2) * norm(y_tilde) * Vo;

    traceWWo = trace(Wo' * Wo);
    traceVVo = trace(Vo' * Vo);

end

== matlab function ImpMinJerkTraj/Sliding Surface1 ==
  data: e_tilde1 input; r_hat output; e_tilde2 input; Lambda1 output; e_tilde3 input; Lambda2 output; Lambda3 output
function [r_hat, Lambda1, Lambda2, Lambda3] = SlidingSurface(e_tilde1, e_tilde2, e_tilde3)

    Lambda1 = 5; Lambda2 = 5; Lambda3 = 5;

    r_hat1  = [Lambda1, 1] * e_tilde1;
    r_hat2  = [Lambda2, 1] * e_tilde2;
    r_hat3  = [Lambda3, 1] * e_tilde3;

    r_hat   = [r_hat1; r_hat2; r_hat3];
    
end

== matlab function ImpMinJerkTraj/MATLAB Function ==
  data: dq input; u input; u_f output; t input; rho output; delta output
function [u_f, rho, delta] = fcn(dq, u, t)

    t01    = 10;
    rho1   = 0.73 + 0.27 * exp(-0.05 * (t-t01)) - 0.13 * tanh(abs(dq(1)) / 1.5);
    delta1 = -0.45 * tanh(dq(1)) - 0.17 * dq(1);

    t02    = 15;
    rho2   = 0.75 + 0.25 * exp(-0.05 * (t-t02)) - 0.08 * tanh(abs(dq(2)) / 2.5);
    delta2 = 0.64 * tanh(dq(2)) - 0.21 * dq(2);

    t03    = 20;
    rho3   = 0.80 + 0.20 * exp(-0.05 * (t-t03)) + 0.15 * tanh(abs(dq(3)) / 0.95);
    delta3 = - 0.71 * tanh(dq(3)) - 0.32 * dq(3);

    u_f = zeros(3, 1);

    if t < t01
        u_f(1) = u(1);
    else
        u_f(1) = rho1 * u(1) + delta1;
    end

    if t < t02
        u_f(2) = u(2);
    else
        u_f(2) = rho2 * u(2) + delta2;
    end

    if t < t03
        u_f(3) = u(3);
    else
        u_f(3) = rho3 * u(3) + delta3;
    end

    rho   = [rho1; rho2; rho3];
    delta = [delta1; delta2; delta3];


end

== matlab function ImpMinJerkTraj/Path Generator ==
  data: t input; q_des output; q_des_f output; dq_des output
function [q_des, q_des_f, dq_des] = PathGen(t)
    
    delay = 700 * 1e-3;
    w = 0.5;
    A = zeros(3, 1);

    q_des   = A *     sin(w*t);
    q_des_f = A *     sin(w*(t + delay));
    dq_des  = A * w * cos(w*t);
    
end
